simulink model "Bebop_sim_spline_faster"  (R2018a)
settings: Solver=VariableStepAuto  StartTime=0.0  StopTime=100  FixedStep=.05  MaxStep=1  MinStep=0.08  RelTol=1  AbsTol=1
values from neighbouring files (symbols this model uses):
  g = 9.81    [initialize_race_no_realtime.m]    (also in initialize_race_realtime.m; initialize_race_realtime_backup_cubic.m; moving_average_rls_own.m = P(i-1)*meas*(lambda+meas*P(i-1)*meas)^-1)
  max_rot_Z = (90)*pi/180    (= 1.57079632679)    [Bebop_sim_init.m]    (also in initialize_race_no_realtime.m = 1.0471975512; initialize_race_realtime.m; initialize_race_realtime_backup_cubic.m; run_batch1.m = list_agility(idx_agility)*max_rot_Z)
  max_theta_X = (40)*pi/180    (= 0.698131700798)    [Bebop_sim_init.m]    (also in initialize_race_no_realtime.m = 0.13962634016; initialize_race_realtime.m = 1.308996939; initialize_race_realtime_backup_cubic.m = 1.308996939; run_batch1.m = list_agility(idx_agility)*max_theta_X)
  max_theta_Y = (40)*pi/180    (= 0.698131700798)    [Bebop_sim_init.m]    (also in initialize_race_no_realtime.m = 0.13962634016; initialize_race_realtime.m = 1.308996939; initialize_race_realtime_backup_cubic.m = 1.308996939; run_batch1.m = list_agility(idx_agility)*max_theta_Y)
  max_v_Z = .5    (= 0.5)    [Bebop_sim_init.m]    (also in initialize_race_no_realtime.m = 1; initialize_race_realtime.m = 3; initialize_race_realtime_backup_cubic.m = 3; run_batch1.m = list_agility(idx_agility)*max_v_Z)
  splines = zeros(3,4,size(gates,1))    [initialize_race_no_realtime.m]    (also in show_splines.m)
  states_num = size(gates_preflight,1)    [initialize_race_no_realtime.m]    (also in initialize_race_realtime.m = size(flightplan,1); initialize_race_realtime_backup_cubic.m = size(flightplan,1))
undefined symbols (not defined in the file or in its folder): fspecial, gray, Rec, SDTV
libraries: sharedtransform x8, simulink x4, visiontextngfix x2, vrlib x2, aerolibutil x1, visionanalysis x1, visiontransforms x1, visionconversions x1
(part 2 of 2)

== matlab function Bebop_sim_spline_faster/select_WP ==
  data: WP_average output; gates input; WP_average input; WP_last output; WP_last input
function [WP_average, WP_last] = select_WP(gates, WP_average, WP_last)
    tVec=zeros(1,3);
    rMat=zeros(3,3);
    
    Resolution = 1*[320, 200];
    vertFOV = 1.05;
    f = 0.5*Resolution(2)/tan(0.5*vertFOV);
    IntrinsicMatrix = [f, 0, 0;
        0, f, 0;
        Resolution/2, 1];
    cameraParams = cameraParameters('IntrinsicMatrix',IntrinsicMatrix); 
    
    %% calculate extrinsics
    worldPoints = size/2*[1 1;
        1 -1;
        -1 1;
        -1 -1];
    
    corners=double(corners);
    if corners == zeros(4,2)
        disp('no corners')
        return
    end
    
    angles = zeros(6,1);
    k = 1;
    for m=1:3
        for n=m+1:4
            angles(k)=atan2(corners(m,2)-corners(n,2),corners(m,1)-corners(n,1));
            k = k+1;            
        end
    end
    angles(angles<=0) = angles(angles<=0)+pi;
    
%     a = zeros(2,1);
%     a = hist(angles,unique(angles));
%     if max(a)>2
%         disp('three occurences')
%         return
%     end
%     
%     
%     
    angles = zeros(2,1);
    angles(1)=atan2(corners(1,2)-corners(4,2),corners(1,1)-corners(4,1));
    angles(2)=atan2(corners(2,2)-corners(3,2),corners(2,1)-corners(3,1));
    angles(angles<=0) = angles(angles<=0)+pi;
    
    if ~(isequal(unique(angles),sort(angles)))
        temp = corners(3,:);
        corners(3,:) = corners(4,:);
        corners(4,:) = temp;
    end
    
    angles(1)=atan2(corners(1,2)-corners(4,2),corners(1,1)-corners(4,1));
    angles(2)=atan2(corners(2,2)-corners(3,2),corners(2,1)-corners(3,1));
    angles(angles<=0) = angles(angles<=0)+pi;
    
    if ~(isequal(unique(angles),sort(angles)))
        corners
        disp('still bad after sort')
        return
    end    
    
    [rMat,tVec] = extrinsics(corners,worldPoints,cameraParams);
%     [orientation,location] = extrinsicsToCameraPose(rMat,tVec);
    
end

== matlab function Bebop_sim_spline_faster/create_spline ==
  data: WP_average input; current_spline output; WP_last input
function current_spline  = create_spline(WP_average, WP_last)
    tVec=zeros(1,3);
    rMat=zeros(3,3);
    
    Resolution = 1*[320, 200];
    vertFOV = 1.05;
    f = 0.5*Resolution(2)/tan(0.5*vertFOV);
    IntrinsicMatrix = [f, 0, 0;
        0, f, 0;
        Resolution/2, 1];
    cameraParams = cameraParameters('IntrinsicMatrix',IntrinsicMatrix); 
    
    %% calculate extrinsics
    worldPoints = size/2*[1 1;
        1 -1;
        -1 1;
        -1 -1];
    
    corners=double(corners);
    if corners == zeros(4,2)
        disp('no corners')
        return
    end
    
    angles = zeros(6,1);
    k = 1;
    for m=1:3
        for n=m+1:4
            angles(k)=atan2(corners(m,2)-corners(n,2),corners(m,1)-corners(n,1));
            k = k+1;            
        end
    end
    angles(angles<=0) = angles(angles<=0)+pi;
    
%     a = zeros(2,1);
%     a = hist(angles,unique(angles));
%     if max(a)>2
%         disp('three occurences')
%         return
%     end
%     
%     
%     
    angles = zeros(2,1);
    angles(1)=atan2(corners(1,2)-corners(4,2),corners(1,1)-corners(4,1));
    angles(2)=atan2(corners(2,2)-corners(3,2),corners(2,1)-corners(3,1));
    angles(angles<=0) = angles(angles<=0)+pi;
    
    if ~(isequal(unique(angles),sort(angles)))
        temp = corners(3,:);
        corners(3,:) = corners(4,:);
        corners(4,:) = temp;
    end
    
    angles(1)=atan2(corners(1,2)-corners(4,2),corners(1,1)-corners(4,1));
    angles(2)=atan2(corners(2,2)-corners(3,2),corners(2,1)-corners(3,1));
    angles(angles<=0) = angles(angles<=0)+pi;
    
    if ~(isequal(unique(angles),sort(angles)))
        corners
        disp('still bad after sort')
        return
    end    
    
    [rMat,tVec] = extrinsics(corners,worldPoints,cameraParams);
%     [orientation,location] = extrinsicsToCameraPose(rMat,tVec);
    
end

== matlab function Bebop_sim_spline_faster/filter_WP ==
  data: WP_list output; WP_average output; WP_list input; WP_current input; WP_average input
function [WP_list, WP_average] = filter_WP(WP_list, WP_current, WP_average)
    tVec=zeros(1,3);
    rMat=zeros(3,3);
    
    Resolution = 1*[320, 200];
    vertFOV = 1.05;
    f = 0.5*Resolution(2)/tan(0.5*vertFOV);
    IntrinsicMatrix = [f, 0, 0;
        0, f, 0;
        Resolution/2, 1];
    cameraParams = cameraParameters('IntrinsicMatrix',IntrinsicMatrix); 
    
    %% calculate extrinsics
    worldPoints = size/2*[1 1;
        1 -1;
        -1 1;
        -1 -1];
    
    corners=double(corners);
    if corners == zeros(4,2)
        disp('no corners')
        return
    end
    
    angles = zeros(6,1);
    k = 1;
    for m=1:3
        for n=m+1:4
            angles(k)=atan2(corners(m,2)-corners(n,2),corners(m,1)-corners(n,1));
            k = k+1;            
        end
    end
    angles(angles<=0) = angles(angles<=0)+pi;
    
%     a = zeros(2,1);
%     a = hist(angles,unique(angles));
%     if max(a)>2
%         disp('three occurences')
%         return
%     end
%     
%     
%     
    angles = zeros(2,1);
    angles(1)=atan2(corners(1,2)-corners(4,2),corners(1,1)-corners(4,1));
    angles(2)=atan2(corners(2,2)-corners(3,2),corners(2,1)-corners(3,1));
    angles(angles<=0) = angles(angles<=0)+pi;
    
    if ~(isequal(unique(angles),sort(angles)))
        temp = corners(3,:);
        corners(3,:) = corners(4,:);
        corners(4,:) = temp;
    end
    
    angles(1)=atan2(corners(1,2)-corners(4,2),corners(1,1)-corners(4,1));
    angles(2)=atan2(corners(2,2)-corners(3,2),corners(2,1)-corners(3,1));
    angles(angles<=0) = angles(angles<=0)+pi;
    
    if ~(isequal(unique(angles),sort(angles)))
        corners
        disp('still bad after sort')
        return
    end    
    
    [rMat,tVec] = extrinsics(corners,worldPoints,cameraParams);
%     [orientation,location] = extrinsicsToCameraPose(rMat,tVec);
    
end

== matlab function Bebop_sim_spline_faster/state_advancement ==
  data: state_new output; dist_new output; state_old input; dist_new input
function [state_new, dist_new] = state_advancement(state_old, dist_new)
    tVec=zeros(1,3);
    rMat=zeros(3,3);
    
    Resolution = 1*[320, 200];
    vertFOV = 1.05;
    f = 0.5*Resolution(2)/tan(0.5*vertFOV);
    IntrinsicMatrix = [f, 0, 0;
        0, f, 0;
        Resolution/2, 1];
    cameraParams = cameraParameters('IntrinsicMatrix',IntrinsicMatrix); 
    
    %% calculate extrinsics
    worldPoints = size/2*[1 1;
        1 -1;
        -1 1;
        -1 -1];
    
    corners=double(corners);
    if corners == zeros(4,2)
        disp('no corners')
        return
    end
    
    angles = zeros(6,1);
    k = 1;
    for m=1:3
        for n=m+1:4
            angles(k)=atan2(corners(m,2)-corners(n,2),corners(m,1)-corners(n,1));
            k = k+1;            
        end
    end
    angles(angles<=0) = angles(angles<=0)+pi;
    
%     a = zeros(2,1);
%     a = hist(angles,unique(angles));
%     if max(a)>2
%         disp('three occurences')
%         return
%     end
%     
%     
%     
    angles = zeros(2,1);
    angles(1)=atan2(corners(1,2)-corners(4,2),corners(1,1)-corners(4,1));
    angles(2)=atan2(corners(2,2)-corners(3,2),corners(2,1)-corners(3,1));
    angles(angles<=0) = angles(angles<=0)+pi;
    
    if ~(isequal(unique(angles),sort(angles)))
        temp = corners(3,:);
        corners(3,:) = corners(4,:);
        corners(4,:) = temp;
    end
    
    angles(1)=atan2(corners(1,2)-corners(4,2),corners(1,1)-corners(4,1));
    angles(2)=atan2(corners(2,2)-corners(3,2),corners(2,1)-corners(3,1));
    angles(angles<=0) = angles(angles<=0)+pi;
    
    if ~(isequal(unique(angles),sort(angles)))
        corners
        disp('still bad after sort')
        return
    end    
    
    [rMat,tVec] = extrinsics(corners,worldPoints,cameraParams);
%     [orientation,location] = extrinsicsToCameraPose(rMat,tVec);
    
end
